simulink model "example_WeatherDatafile"  (R2018b)
settings: Solver=ode45  StartTime=0.0  StopTime=365*24*3600  RelTol=1e-3  EnableMultiTasking=on
undefined symbols (not defined in the file): path_carnot
libraries: carnot x1
settings Model: Creator=drhf  LastModifiedBy=drhf
settings DataIOCC: LimitDataPoints=on  SaveFormat=Array
settings OptimizationCC: ExpressionDepthLimit=2147483647  LifeSpan=inf
settings DebuggingCC: UnderspecifiedInitializationDetection=Classic  MergeDetectMultiDrivingBlocksExec=none  StateNameClashWarn=warning  SFUnexpectedBacktrackingDiag=warning  SFNoUnconditionalDefaultTransitionDiag=warning  SFExecutionAtInitializationDiag=none
settings HardwareCC: ProdBitPerPointer=32  ProdBitPerSizeT=32  ProdBitPerPtrDiffT=32  ProdLargestAtomicFloat=None  ProdIntDivRoundTo=Undefined  ProdEndianess=Unspecified  ProdWordSize=32  ProdHWDeviceType=32-bit Generic
settings ModelReferenceCC: PropagateSignalLabelsOutOfModel=off
settings SFSimCC: SimUseLocalCustomCode=off
settings RTWCC: RTWUseLocalCustomCode=off
settings CodeAppCC: StateflowObjectComments=on
settings GRTTargetCC: TargetLangStandard=C89/C90 (ANSI)  GeneratePreprocessorConditionals=Disable all  CombineOutputUpdateFcns=off  GRTInterface=on
settings ConfigComp: CovMetricSettings=dw  CovHtmlReporting=on  CovSaveCumulativeToWorkspaceVar=on  CovSaveSingleToWorkspaceVar=on  CovExternalEMLEnable=off

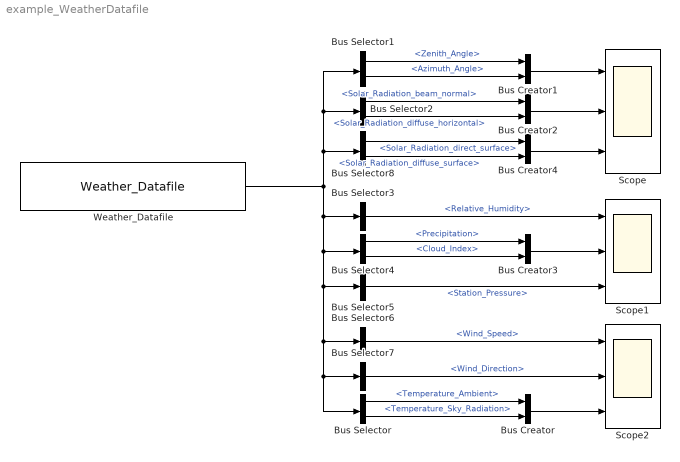
== system example_WeatherDatafile ==
  Bus Creator{,1..4} (5 alike) : BusCreator  Inputs=2
  Bus Selector : BusSelector  OutputSignals=Temperature_Ambient,Temperature_Sky_Radiation
  Bus Selector1 : BusSelector  OutputSignals=Zenith_Angle,Azimuth_Angle
  Bus Selector2 : BusSelector  OutputSignals=Solar_Radiation_beam_normal,Solar_Radiation_diffuse_horizontal
  Bus Selector3 : BusSelector  OutputSignals=Relative_Humidity
  Bus Selector4 : BusSelector  OutputSignals=Precipitation,Cloud_Index
  Bus Selector5 : BusSelector  OutputSignals=Station_Pressure
  Bus Selector6 : BusSelector  OutputSignals=Wind_Speed
  Bus Selector7 : BusSelector  OutputSignals=Wind_Direction
  Bus Selector8 : BusSelector  OutputSignals=Solar_Radiation_direct_surface,Solar_Radiation_diffuse_surface
  Scope : Scope  NumInputPorts=3
  Scope1 : Scope  NumInputPorts=3
  Scope2 : Scope  NumInputPorts=3
  Weather_Datafile : carnot/Weather/Weather_Datafile  PathName=path_carnot('data')  FileName='DE_TRY2016_Potsdam_averageYear.mat'  UserParam=off  VariableName=DE_TRY2010_01_extremeWinter  SampleTime=3600
      settings: SourceProductName=Carnot
  wires:
  Weather_Datafile/1 -> Bus Selector/1, Bus Selector7/1, Bus Selector6/1, Bus Selector5/1, Bus Selector4/1, Bus Selector3/1, Bus Selector1/1, Bus Selector2/1, Bus Selector8/1
  Bus Creator1/1 -> Scope/1
  Bus Selector3/1 -> Scope1/1  "<Relative_Humidity>"
  Bus Selector5/1 -> Scope1/3  "<Station_Pressure>"
  Bus Selector6/1 -> Scope2/1  "<Wind_Speed>"
  Bus Selector7/1 -> Scope2/2  "<Wind_Direction>"
  Bus Selector/1 -> Bus Creator/1  "<Temperature_Ambient>"
  Bus Selector/2 -> Bus Creator/2  "<Temperature_Sky_Radiation>"
  Bus Selector1/1 -> Bus Creator1/1  "<Zenith_Angle>"
  Bus Selector1/2 -> Bus Creator1/2  "<Azimuth_Angle>"
  Bus Creator2/1 -> Scope/2
  Bus Selector2/1 -> Bus Creator2/1  "<Solar_Radiation_beam_normal>"
  Bus Selector2/2 -> Bus Creator2/2  "<Solar_Radiation_diffuse_horizontal>"
  Bus Creator3/1 -> Scope1/2
  Bus Selector4/1 -> Bus Creator3/1  "<Precipitation>"
  Bus Selector4/2 -> Bus Creator3/2  "<Cloud_Index>"
  Bus Creator/1 -> Scope2/3
  Bus Selector8/1 -> Bus Creator4/1  "<Solar_Radiation_direct_surface>"
  Bus Selector8/2 -> Bus Creator4/2  "<Solar_Radiation_diffuse_surface>"
  Bus Creator4/1 -> Scope/3
